simulink model "PID_Loop_2023a"  (R2023a)
settings: Solver=FixedStepAuto  StartTime=0.0  StopTime=tspan  FixedStep=dt  RelTol=1e-3
model workspace (MAT data in the model file):
  Drag_Constants = 1
  mass = [5.51 5.51 5.51 1 1 1]
  mass_6a = [5 5 5 1 1 1]
values from neighbouring files (symbols this model uses):
  do_bouyancy_flag = 1    [PID_testing_data_producer.m]    (also in init.m = 0)
  do_drag_flag = 1    [PID_testing_data_producer.m]
  do_gravity_flag = 1    [PID_testing_data_producer.m]    (also in init.m = 0)
  drag_wrench = [ ... (first row only)    [constants.m]    (also in constants.mat = [0.41 0 0 0 0 0 0 0.5 0 0 0 0 ... (36 elements, 6x6)])
  dt = 0.001    [PID_testing_data_producer.m]    (also in init.m)
  Dt = 0.01    [init.m]
  dt_controller = 0.01    [PID_testing_data_producer.m]
  dt_filter = 0.01    [PID_testing_data_producer.m]    (also in init.m)
  dt_imu = 0.01    [PID_testing_data_producer.m]
  dt_plotting = 0.01    [PID_testing_data_producer.m]
  g = 9.8067    [constants.m]    (also in constants.mat = 9.80665)
  H = [1 0 0 ... (first row only)    [init.m]
  inverse_wrench = pinv(wrench)    [calculate_wrench.m]    (also in constants.m = geometry_properties.inverse_wrench; geometry_properties.mat = [0.09 0.09 -0.09 -0.09 0.353553390593 0.353553390593 0.35355)
  max_pitch_torque = norm(wrench*(F_max*[1 1 -1 -1 0 0 0 0]'))    [calculate_wrench.m]
  max_roll_torque = norm(wrench*(F_max*[1 -1 1 -1 0 0 0 0]'))    [calculate_wrench.m]
  max_yaw_torque = norm(wrench*(F_max*[0 0 0 0 -1 1 -1 1]'))    [calculate_wrench.m]
  OperatingVoltage = Voltage    (= 16)    [constants.m]
  Q = diag([0.0001, 0.0001, 0.1])    [init.m]
  R = [.1 0 ... (first row only)    [init.m]
  states_desired = [x_des;E_des]    [init.m]
  v0_e = [0,0,0]'    [PID_testing_data_producer.m]    (also in init.m = [pi/6, -pi/6, pi]')
  Voltage = 16    [constants.m]
  volume = 0.0074    [constants.m]    (also in constants.mat = 0.0073741788)
  volume_center = [0, 0, -0.07]    [constants.m]    (also in constants.mat = [0 0 0.1])
  water_density = 997    [constants.m]    (also in constants.mat = 1000)
  waypoints = input_state_errors(:,i)    [PID_testing_data_producer.m]    (also in init.m = [0, 0, 0])
  wrench = eval(w)    [calculate_wrench.m]    (also in constants.m = geometry_properties.wrench; constants.mat = [0 0 0 0 -0.7071 -0.7071 -0.7071 -0.7071 0 0 0 0 ... (48 ele; geometry_properties.mat = [0 0 -1 0.22 0.25 0 0 0 -1 -0.22 0.25 0 ... (48 elements, 6x; wrench.m)
  x0_e = [0,0,0]'    [PID_testing_data_producer.m]    (also in init.m = [0, 0, 0]')
undefined symbols (not defined in the file or in its folder): IMU, P, Zero_Time
libraries: slpidlib x4, shared6dof x1, mspfiltlib x1, dspstat3 x1, mspsensorlib x1
(part 1 of 2)
settings Model: Creator=zenyn  LastModifiedBy=zafak
settings DataIOCC: LoggingToFile=on
settings OptimizationCC: EnhancedBackFolding=on  PassReuseOutputArgsAs=Individual arguments  ZeroExternalMemoryAtStartup=off  ZeroInternalMemoryAtStartup=off  MaxStackSize=64  OptimizeBlockOrder=speed  DifferentSizesBufferReuse=on  OptimizationCustomize=off  EfficientTunableParamExpr=on
settings DebuggingCC: ParameterTunabilityLossMsg=error
settings SFSimCC: MATLABDynamicMemAlloc=off
settings RTWCC: Description=Embedded Coder  SystemTargetFile=ert.tlc  HardwareBoard=Robot Operating System 2 (ROS 2)  TLCOptions="-aInlineSetEventsForThisBaseRateFcn=TLC_FALSE -aSuppressMultiTaskScheduler=TLC_FALSE  -aRateBasedStepFcn=0"  TemplateMakefile=ert_default_tmf  Toolchain=Colcon Tools  TargetLang=C++  GPUComputeCapability=5.0
settings CodeAppCC: ForceParamTrailComments=on  IgnoreCustomStorageClasses=off  OperatorAnnotations=on  SimulinkDataObjDesc=on  SFDataObjDesc=on  InsertBlockDesc=on
settings ERTTargetCC: CodeInterfacePackaging=C++ class  RootIOFormat=Structure reference

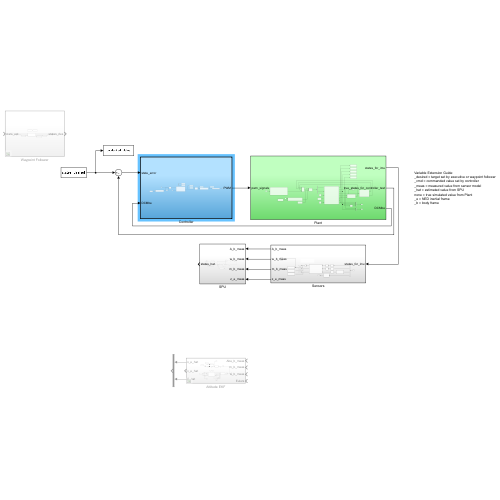
[thumbnail: Simulink's stored preview of the top-level diagram]
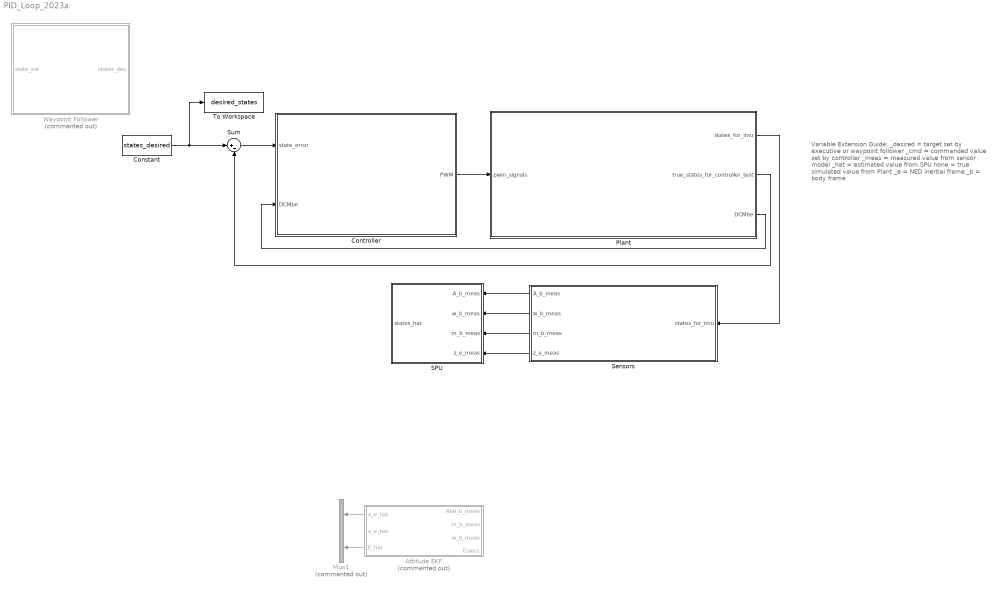
== system PID_Loop_2023a ==
  note: Variable Extension Guide:
      | _desired = target set by executive or waypoint follower
      | _cmd = commanded value set by controller
      | _meas = measured value from sensor model
      | _hat = estimated value from SPU
      | none = true simulated value from Plant
      | _e = NED inertial frame
      | _b = body frame
  Attitude EKF : Subsystem  Commented=on
  Constant : Constant  Value=states_desired
  Controller : Subsystem  TreatAsAtomicUnit=on
  Mux1 : Mux  Commented=on  Inputs=2
  Plant : Subsystem
  SPU : Subsystem
  Sensors : Subsystem
  Sum : Sum  Inputs=|+-
  To Workspace : ToWorkspace  VariableName=desired_states  SaveFormat=Timeseries  SampleTime=dt_plotting
  Waypoint Follower : Subsystem  Commented=on
  wires:
  Constant/1 -> Sum/1, To Workspace/1
  Sum/1 -> Controller/1(state_error)
  Controller/1(PWM) -> Plant/1(pwm_signals)
  Plant/2(true_states_for_controller_test) -> Sum/2
  Attitude EKF/1(x_e_hat) -> Mux1/1
  Attitude EKF/3(E_hat) -> Mux1/2
  Plant/1(states_for_imu) -> Sensors/1(states_for_imu)
  Sensors/1(A_b_meas) -> SPU/1(A_b_meas)
  Sensors/2(w_b_meas) -> SPU/2(w_b_meas)
  Sensors/3(m_b_meas) -> SPU/3(m_b_meas)
  Plant/3(DCMbe) -> Controller/2(DCMbe)
  Sensors/4(z_e_meas) -> SPU/4(z_e_meas)

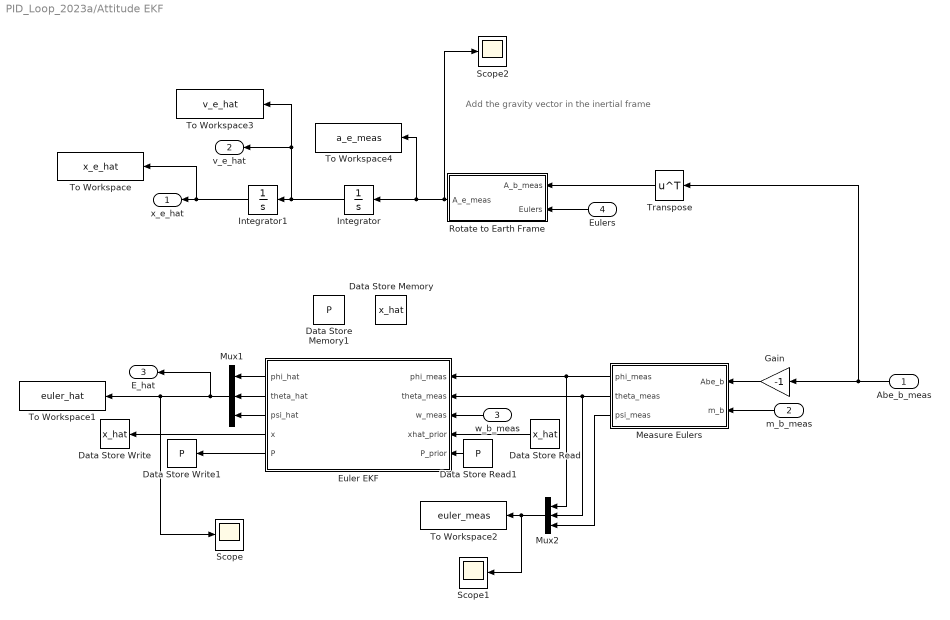
== system PID_Loop_2023a/Attitude EKF ==
  note: Add the gravity vector in the inertial frame
  Abe_b_meas : Inport  SampleTime=dt_filter
  m_b_meas : Inport  Port=2  SampleTime=dt_filter
  w_b_meas : Inport  Port=3
  Eulers : Inport  Port=4
  Data Store Memory : DataStoreMemory  DataStoreName=x_hat  WriteAfterWriteMsg=warning  InitialValue=xhat0  ShowAdditionalParam=off
  Data Store Memory1 : DataStoreMemory  DataStoreName=P  WriteAfterWriteMsg=warning  InitialValue=P0  ShowAdditionalParam=off
  Data Store Read : DataStoreRead  DataStoreName=x_hat  IndexOptions=Index vector (dialog)  Indices=1  OutputSizes=1
  Data Store Read1 : DataStoreRead  DataStoreName=P  IndexOptions=Index vector (dialog)  Indices=1  OutputSizes=1
  Data Store Write : DataStoreWrite  DataStoreName=x_hat  IndexOptions=Index vector (dialog)  Indices=1  OutputSizes=1
  Data Store Write1 : DataStoreWrite  DataStoreName=P  IndexOptions=Index vector (dialog)  Indices=1  OutputSizes=1
  Euler EKF : MATLAB Function  TreatAsAtomicUnit=on
  Gain : Gain  Gain=-1
  Integrator : Integrator  InitialCondition=v0_e
  Integrator1 : Integrator  InitialCondition=x0_e
  Measure Eulers : MATLAB Function  TreatAsAtomicUnit=on
  Mux1 : Mux  Inputs=3
  Mux2 : Mux  Inputs=3
  Rotate to Earth Frame : MATLAB Function  TreatAsAtomicUnit=on
  Scope : Scope
  Scope1 : Scope
  Scope2 : Scope
  To Workspace : ToWorkspace  VariableName=x_e_hat  SaveFormat=Timeseries  SampleTime=dt_plotting
  To Workspace1 : ToWorkspace  VariableName=euler_hat  SaveFormat=Timeseries  SampleTime=dt_plotting
  To Workspace2 : ToWorkspace  VariableName=euler_meas  SaveFormat=Timeseries  SampleTime=dt_plotting
  To Workspace3 : ToWorkspace  VariableName=v_e_hat  SaveFormat=Timeseries  SampleTime=dt_plotting
  To Workspace4 : ToWorkspace  VariableName=a_e_meas  SaveFormat=Timeseries  SampleTime=-1
  Transpose : Math  Operator=transpose
  x_e_hat : Outport
  v_e_hat : Outport  Port=2
  E_hat : Outport  Port=3
  wires:
  Measure Eulers/1(phi_meas) -> Euler EKF/1(phi_meas), Mux2/1
  Euler EKF/4(x) -> Data Store Write/1
  Measure Eulers/2(theta_meas) -> Mux2/2, Euler EKF/2(theta_meas)
  Mux1/1 -> E_hat/1, Scope/1, To Workspace1/1
  Data Store Read1/1 -> Euler EKF/5(P_prior)
  Euler EKF/1(phi_hat) -> Mux1/1
  Euler EKF/5(P) -> Data Store Write1/1
  Euler EKF/3(psi_hat) -> Mux1/3
  Euler EKF/2(theta_hat) -> Mux1/2
  Data Store Read/1 -> Euler EKF/4(xhat_prior)
  Abe_b_meas/1 -> Gain/1, Transpose/1
  Measure Eulers/3(psi_meas) -> Mux2/3
  Mux2/1 -> Scope1/1, To Workspace2/1
  m_b_meas/1 -> Measure Eulers/2(m_b)
  w_b_meas/1 -> Euler EKF/3(w_meas)
  Integrator/1 -> To Workspace3/1, v_e_hat/1, Integrator1/1
  Integrator1/1 -> To Workspace/1, x_e_hat/1
  Gain/1 -> Measure Eulers/1(Abe_b)
  Rotate to Earth Frame/1(A_e_meas) -> Scope2/1, To Workspace4/1, Integrator/1
  Eulers/1 -> Rotate to Earth Frame/2(Eulers)
  Transpose/1 -> Rotate to Earth Frame/1(A_b_meas)

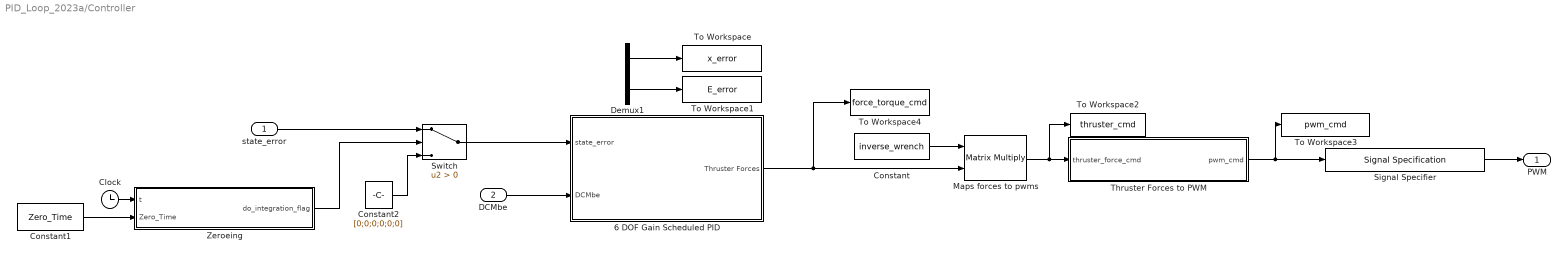
== system PID_Loop_2023a/Controller ==
  state_error : Inport  SampleTime=dt_controller
  DCMbe : Inport  Port=2
  6 DOF Gain Scheduled PID : Subsystem
  Clock : Clock
  Constant : Constant  Value=inverse_wrench
  Constant1 : Constant  Value=Zero_Time
  Constant2 : Constant  Value=[0;0;0;0;0;0]
  Demux1 : Demux  Outputs=2
  Maps forces to pwms : Product  Multiplication=Matrix(*)
  Signal Specifier : SignalSpecification  OutMin=[1200 ]  OutMax=[ 1800 ]  OutDataTypeStr=double  Unit=µs  Dimensions=[8 1]
  Switch : Switch  Criteria=u2 > Threshold  SaturateOnIntegerOverflow=off  InputSameDT=off
  Thruster Forces to PWM : MATLAB Function  TreatAsAtomicUnit=on
  To Workspace : ToWorkspace  VariableName=x_error  SaveFormat=Timeseries  SampleTime=dt_plotting
  To Workspace1 : ToWorkspace  VariableName=E_error  SaveFormat=Timeseries  SampleTime=dt_plotting
  To Workspace2 : ToWorkspace  VariableName=thruster_cmd  SaveFormat=Timeseries  SampleTime=dt_plotting
  To Workspace3 : ToWorkspace  VariableName=pwm_cmd  SaveFormat=Timeseries  SampleTime=dt_plotting
  To Workspace4 : ToWorkspace  VariableName=force_torque_cmd  SaveFormat=Timeseries  SampleTime=dt_plotting
  Zeroeing : MATLAB Function  TreatAsAtomicUnit=on
  PWM : Outport
  wires:
  Thruster Forces to PWM/1(pwm_cmd) -> Signal Specifier/1, To Workspace3/1
  Signal Specifier/1 -> PWM/1
  Demux1/1 -> To Workspace/1
  Demux1/2 -> To Workspace1/1
  Maps forces to pwms/1 -> Thruster Forces to PWM/1(thruster_force_cmd), To Workspace2/1
  Constant/1 -> Maps forces to pwms/1
  6 DOF Gain Scheduled PID/1(Thruster Forces) -> To Workspace4/1, Maps forces to pwms/2
  DCMbe/1 -> 6 DOF Gain Scheduled PID/2(DCMbe)
  Clock/1 -> Zeroeing/1(t)
  Constant1/1 -> Zeroeing/2(Zero_Time)
  Switch/1 -> 6 DOF Gain Scheduled PID/1(state_error)
  state_error/1 -> Switch/1
  Zeroeing/1(do_integration_flag) -> Switch/2
  Constant2/1 -> Switch/3

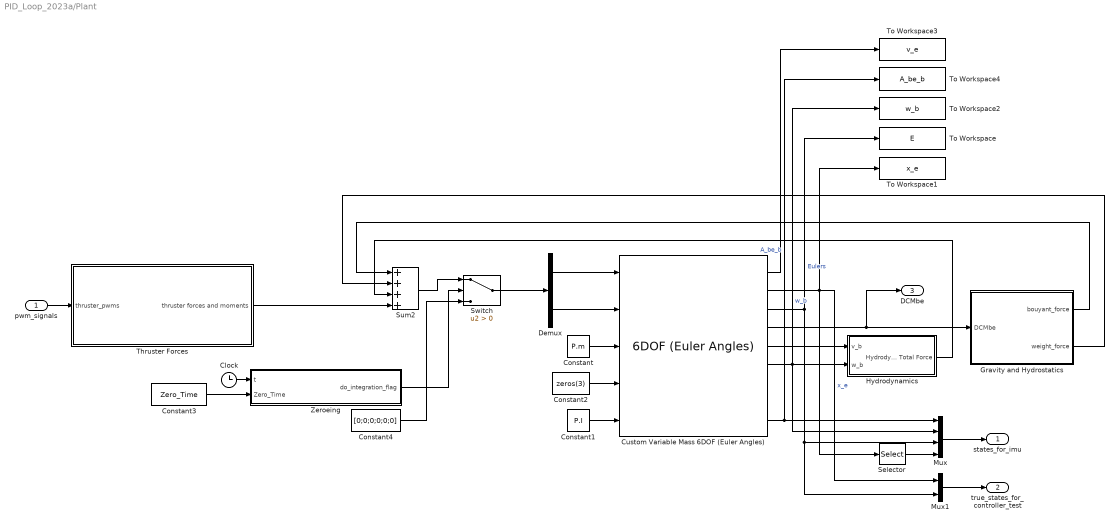
== system PID_Loop_2023a/Plant ==
  pwm_signals : Inport  SampleTime=dt
  Clock : Clock
  Constant : Constant  Value=P.m
  Constant1 : Constant  Value=P.I
  Constant2 : Constant  Value=zeros(3)
  Constant3 : Constant  Value=Zero_Time
  Constant4 : Constant  Value=[0;0;0;0;0;0]
  Custom Variable Mass 6DOF (Euler Angles) : shared6dof/6DOF (Euler Angles)  units=Metric (MKS)  mtype=Custom Variable  rep=Euler Angles  xme_0=x0_e  Vm_0=v0_e  eul_0=E0  pm_0=w0  mass_0=1.0  mass_e=0.5  mass_f=2.0  inertia=eye(3)  inertia_e=eye(3)  inertia_f=2*eye(3)  k_quat=1.0  vre_flag=off  abi_flag=on  aMode=0  xme_statename=''  Vm_statename=''  eul_statename=''  quat_statename=''  pm_statename=''  mass_statename=''
      settings: LibrarySourceBlock=aerolib6dof2/Custom Variable Mass 6DOF (Euler Angles)
  Demux : Demux  Outputs=2
  Gravity and Hydrostatics : Subsystem
  Hydrodynamics : Subsystem
  Mux : Mux
  Mux1 : Mux  Inputs=2
  Selector : Selector  InputPortWidth=3  IndexOptions=Index vector (dialog)  Indices=[3]  OutputSizes=1
  Sum2 : Sum  Inputs=++++
  Switch : Switch  Criteria=u2 > Threshold  SaturateOnIntegerOverflow=off  InputSameDT=off
  Thruster Forces : Subsystem
  To Workspace : ToWorkspace  VariableName=E  SaveFormat=Timeseries  SampleTime=dt_plotting
  To Workspace1 : ToWorkspace  VariableName=x_e  SaveFormat=Timeseries  SampleTime=dt_plotting
  To Workspace2 : ToWorkspace  VariableName=w_b  SaveFormat=Timeseries  SampleTime=dt_plotting
  To Workspace3 : ToWorkspace  VariableName=v_e  SaveFormat=Timeseries  SampleTime=dt_plotting
  To Workspace4 : ToWorkspace  VariableName=A_be_b  SaveFormat=Timeseries  SampleTime=dt_plotting
  Zeroeing : MATLAB Function  TreatAsAtomicUnit=on
  states_for_imu : Outport
  true_states_for_controller_test : Outport  Port=2
  DCMbe : Outport  Port=3
  wires:
  Constant/1 -> Custom Variable Mass 6DOF (Euler Angles)/3
  Constant1/1 -> Custom Variable Mass 6DOF (Euler Angles)/5
  Constant2/1 -> Custom Variable Mass 6DOF (Euler Angles)/4
  pwm_signals/1 -> Thruster Forces/1(thruster_pwms)
  Gravity and Hydrostatics/2(weight_force) -> Sum2/2
  Demux/2 -> Custom Variable Mass 6DOF (Euler Angles)/2
  Demux/1 -> Custom Variable Mass 6DOF (Euler Angles)/1
  Gravity and Hydrostatics/1(bouyant_force) -> Sum2/1
  Hydrodynamics/1(Hydrodynamic Total Force) -> Sum2/3
  Mux/1 -> states_for_imu/1
  Mux1/1 -> true_states_for_controller_test/1
  Custom Variable Mass 6DOF (Euler Angles)/4 -> DCMbe/1, Gravity and Hydrostatics/1(DCMbe)
  Custom Variable Mass 6DOF (Euler Angles)/5 -> Hydrodynamics/1(v_b)
  Custom Variable Mass 6DOF (Euler Angles)/6 -> Hydrodynamics/2(w_b), Mux/2, To Workspace2/1  "w_b"
  Custom Variable Mass 6DOF (Euler Angles)/9 -> To Workspace4/1, Mux/1  "A_be_b"
  Custom Variable Mass 6DOF (Euler Angles)/3 -> To Workspace/1, Mux1/2, Mux/3  "Eulers"
  Custom Variable Mass 6DOF (Euler Angles)/1 -> To Workspace3/1
  Thruster Forces/1(thruster forces and moments) -> Sum2/4
  Clock/1 -> Zeroeing/1(t)
  Constant3/1 -> Zeroeing/2(Zero_Time)
  Constant4/1 -> Switch/3
  Custom Variable Mass 6DOF (Euler Angles)/2 -> Mux1/1, Selector/1, To Workspace1/1  "x_e"
  Selector/1 -> Mux/4
  Sum2/1 -> Switch/1
  Switch/1 -> Demux/1
  Zeroeing/1(do_integration_flag) -> Switch/2

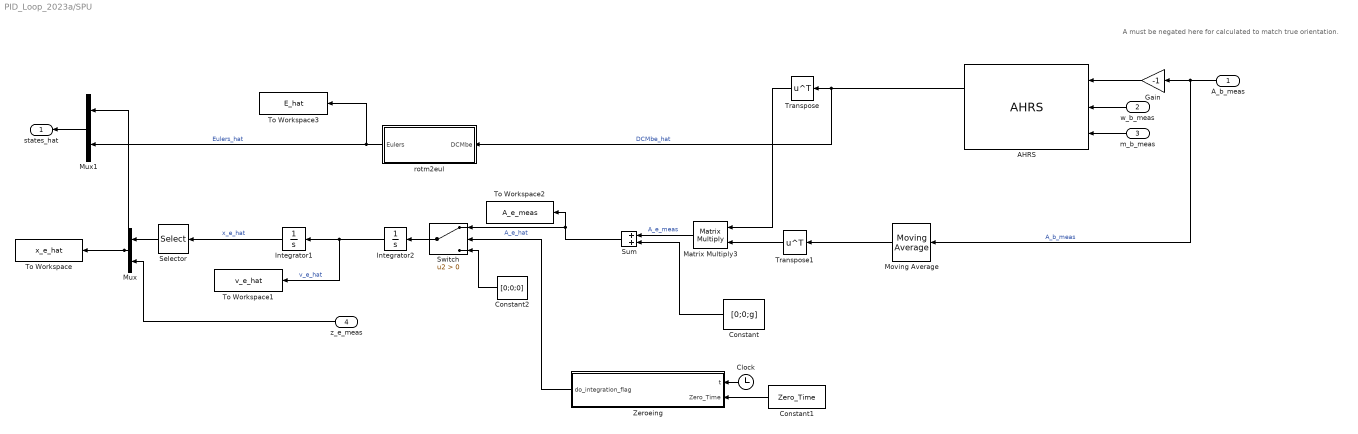
== system PID_Loop_2023a/SPU ==
  note: A must be negated here for calculated to match true orientation.
  A_b_meas : Inport  SampleTime=dt_filter
  w_b_meas : Inport  Port=2  SampleTime=dt_filter
  m_b_meas : Inport  Port=3  SampleTime=dt_filter
  z_e_meas : Inport  Port=4
  AHRS : mspfiltlib/AHRS  DispRefFrame=NED  DecimationFactor=1  InitialProcessNoise=ahrsfilter.defaultProcessNoise  OrientationFormat=Rotation matrix  SimulateUsing=Interpreted execution  AccelerometerNoise=AHRS.accel_noise  GyroscopeNoise=AHRS.gyro_noise  MagnetometerNoise=AHRS.mag_noise  GyroscopeDriftNoise=AHRS.gyro_drift_noise  LinearAccelerationNoise=AHRS.env_lin_accel_noise  MagneticDisturbanceNoise=AHRS.env_mag_disturbance_noise  LinearAccelerationDecayFactor=AHRS.env_lin_accel_decay_factor  MagneticDisturbanceDecayFactor=AHRS.env_mag_disturbance_decay_factor  ExpectedMagneticFieldStrength=AHRS.env_mag_field_strength
  Clock : Clock
  Constant : Constant  Value=[0;0;g]
  Constant1 : Constant  Value=Zero_Time
  Constant2 : Constant  Value=[0;0;0]
  Gain : Gain  Gain=-1
  Integrator1 : Integrator  InitialCondition=x0_e
  Integrator2 : Integrator  InitialCondition=v0_e
  Matrix Multiply3 : Product  Multiplication=Matrix(*)
  Moving Average : dspstat3/Moving Average  Method=Sliding window  ForgettingFactorPort=off  SpecifyWindowLength=on  WindowLength=10  OverlapLength=9  AllowArbitraryInputLength=off  ForgettingFactor=0.9  SimulateUsing=Code generation
  Mux : Mux  Inputs=2
  Mux1 : Mux  Inputs=2
  Selector : Selector  InputPortWidth=3  IndexOptions=Index vector (dialog)  Indices=[1 2]  OutputSizes=1
  Sum : Sum
  Switch : Switch  Criteria=u2 > Threshold  SaturateOnIntegerOverflow=off  InputSameDT=off
  To Workspace : ToWorkspace  VariableName=x_e_hat  SaveFormat=Timeseries  SampleTime=dt_plotting
  To Workspace1 : ToWorkspace  VariableName=v_e_hat  SaveFormat=Timeseries  SampleTime=dt_plotting
  To Workspace2 : ToWorkspace  VariableName=A_e_meas  SaveFormat=Timeseries  SampleTime=-1
  To Workspace3 : ToWorkspace  VariableName=E_hat  SaveFormat=Timeseries  SampleTime=-1
  Transpose : Math  Operator=transpose
  Transpose1 : Math  Operator=transpose
  Zeroeing : MATLAB Function  TreatAsAtomicUnit=on
  rotm2eul : MATLAB Function  TreatAsAtomicUnit=on
  states_hat : Outport
  wires:
  Mux/1 -> To Workspace/1, Mux1/1
  A_b_meas/1 -> Moving Average/1, Gain/1  "A_b_meas"
  Integrator2/1 -> To Workspace1/1, Integrator1/1  "v_e_hat"
  m_b_meas/1 -> AHRS/3
  AHRS/1 -> rotm2eul/1(DCMbe), Transpose/1  "DCMbe_hat"
  w_b_meas/1 -> AHRS/2
  Transpose/1 -> Matrix Multiply3/1
  Mux1/1 -> states_hat/1
  rotm2eul/1(Eulers) -> To Workspace3/1, Mux1/2  "Eulers_hat"
  Gain/1 -> AHRS/1
  Matrix Multiply3/1 -> Sum/1  "A_e_meas"
  Constant/1 -> Sum/2
  Transpose1/1 -> Matrix Multiply3/2
  Moving Average/1 -> Transpose1/1
  Clock/1 -> Zeroeing/1(t)
  Constant1/1 -> Zeroeing/2(Zero_Time)
  Constant2/1 -> Switch/3
  Integrator1/1 -> Selector/1  "x_e_hat"
  Selector/1 -> Mux/1
  Sum/1 -> To Workspace2/1, Switch/1  "A_e_hat"
  Switch/1 -> Integrator2/1
  z_e_meas/1 -> Mux/2
  Zeroeing/1(do_integration_flag) -> Switch/2

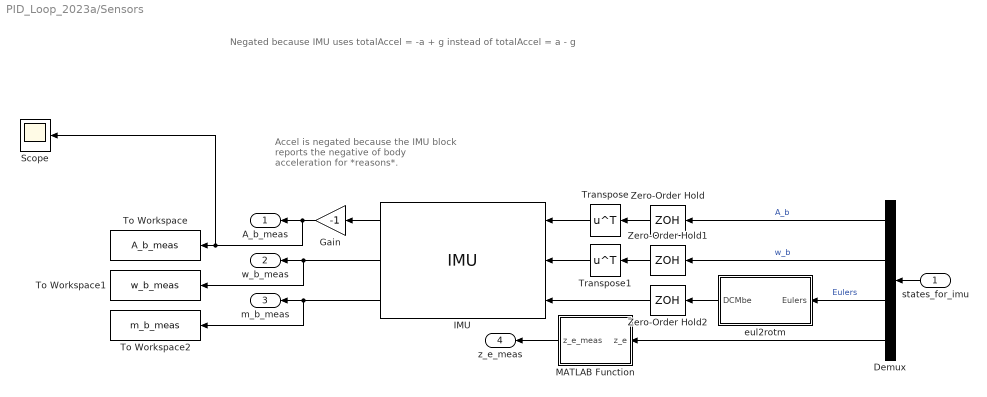
== system PID_Loop_2023a/Sensors ==
  note: Accel is negated because the IMU block reports the negative of body acceleration for *reasons*.
  note: Negated because IMU uses totalAccel = -a + g instead of totalAccel = a - g
  states_for_imu : Inport  SampleTime=dt_imu
  Demux : Demux  Outputs=[3,3,3,1]
  Gain : Gain  Gain=-1
  IMU : mspsensorlib/IMU  DispRefFrame=NED  Temperature=25  MagneticFieldNED=[27.550, -2.4169, -16]  MagneticFieldENU=[ -2.4169, 27.5550, 16.0849 ]  SeedDouble=102  SimulateUsing=Interpreted execution  AccelParamsMeasurementRange=IMU.accelMaxRating  AccelParamsResolution=0  AccelParamsConstantBias=[ 0, 0, 0 ]  AccelParamsAxesMisalignment=[ 100, 0, 0; 0, 100, 0; 0, 0, 100 ]  AccelParamsNoiseDensity=IMU.accelVelRNDWalk*[ 1, 1, 1 ]  AccelParamsBiasInstability=IMU.accelBiasInstability*[ 1, 1, 1 ]  AccelParamsRandomWalk=IMU.accelAccelRNDWalk*[1, 1, 1]  AccelParamsTemperatureBias=[ 0, 0, 0 ]  AccelParamsTemperatureScaleFactor=[ 0, 0, 0 ]  GyroParamsMeasurementRange=Inf  GyroParamsResolution=0  GyroParamsConstantBias=[ 0, 0, 0 ]  GyroParamsAxesMisalignment=[ 100, 0, 0; 0, 100, 0; 0, 0, 100 ]  GyroParamsAccelerationBias=[ 0, 0, 0 ]  GyroParamsNoiseDensity=IMU.gyroAngleRNDWalk*[ 1, 1, 1 ]  GyroParamsBiasInstability=IMU.gyroBiasInstability*[ 1, 1, 1 ]  GyroParamsRandomWalk=IMU.gyroRateRNDWalk*[1, 1, 1]  GyroParamsTemperatureBias=[ 0, 0, 0 ]  GyroParamsTemperatureScaleFactor=[ 0, 0, 0 ]  MagParamsMeasurementRange=Inf  MagParamsResolution=0  MagParamsConstantBias=[ 0, 0, 0 ]  MagParamsAxesMisalignment=[ 100, 0, 0; 0, 100, 0; 0, 0, 100 ]  MagParamsNoiseDensity=IMU.magsRateRNDWalk*[1, 1, 1]  MagParamsBiasInstability=IMU.magsBiasInstability*[1, 1, 1]  MagParamsRandomWalk=IMU.magsRNDWalk*[1, 1, 1]  MagParamsTemperatureBias=[ 0, 0, 0 ]  MagParamsTemperatureScaleFactor=[ 0, 0, 0 ]
  MATLAB Function : MATLAB Function  TreatAsAtomicUnit=on
  Scope : Scope
  To Workspace : ToWorkspace  VariableName=A_b_meas  SaveFormat=Timeseries  SampleTime=dt_plotting
  To Workspace1 : ToWorkspace  VariableName=w_b_meas  SaveFormat=Timeseries  SampleTime=dt_plotting
  To Workspace2 : ToWorkspace  VariableName=m_b_meas  SaveFormat=Timeseries  SampleTime=dt_plotting
  Transpose : Math  Operator=transpose
  Transpose1 : Math  Operator=transpose
  Zero-Order Hold : ZeroOrderHold  SampleTime=dt_filter
  Zero-Order Hold1 : ZeroOrderHold  SampleTime=dt_filter
  Zero-Order Hold2 : ZeroOrderHold  SampleTime=dt_filter
  eul2rotm : MATLAB Function  TreatAsAtomicUnit=on
  A_b_meas : Outport
  w_b_meas : Outport  Port=2
  m_b_meas : Outport  Port=3
  z_e_meas : Outport  Port=4
  wires:
  Transpose/1 -> IMU/1
  Zero-Order Hold/1 -> Transpose/1
  Transpose1/1 -> IMU/2
  Zero-Order Hold1/1 -> Transpose1/1
  Demux/1 -> Zero-Order Hold/1  "A_b"
  Zero-Order Hold2/1 -> IMU/3
  IMU/2 -> w_b_meas/1, To Workspace1/1
  IMU/3 -> m_b_meas/1, To Workspace2/1
  Demux/2 -> Zero-Order Hold1/1  "w_b"
  IMU/1 -> Gain/1
  Gain/1 -> Scope/1, To Workspace/1, A_b_meas/1
  states_for_imu/1 -> Demux/1
  Demux/3 -> eul2rotm/1(Eulers)  "Eulers"
  eul2rotm/1(DCMbe) -> Zero-Order Hold2/1
  Demux/4 -> MATLAB Function/1(z_e)
  MATLAB Function/1(z_e_meas) -> z_e_meas/1

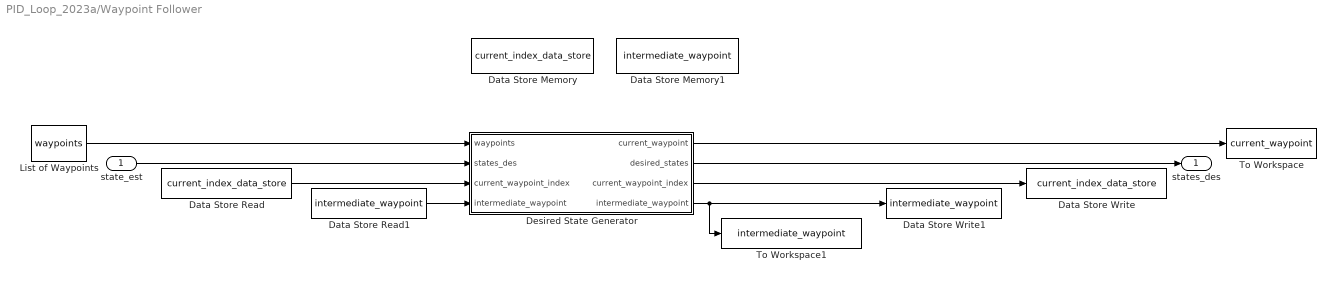
== system PID_Loop_2023a/Waypoint Follower ==
  state_est : Inport  SampleTime=Dt
  Data Store Memory : DataStoreMemory  DataStoreName=current_index_data_store  WriteAfterWriteMsg=warning  InitialValue=1  ShowAdditionalParam=off
  Data Store Memory1 : DataStoreMemory  DataStoreName=intermediate_waypoint  WriteAfterWriteMsg=warning  InitialValue=[9999,9999,9999]  ShowAdditionalParam=off
  Data Store Read : DataStoreRead  DataStoreName=current_index_data_store  IndexOptions=Index vector (dialog)  Indices=1  OutputSizes=1
  Data Store Read1 : DataStoreRead  DataStoreName=intermediate_waypoint  IndexOptions=Index vector (dialog)  Indices=1  OutputSizes=1
  Data Store Write : DataStoreWrite  DataStoreName=current_index_data_store  IndexOptions=Index vector (dialog)  Indices=1  OutputSizes=1
  Data Store Write1 : DataStoreWrite  DataStoreName=intermediate_waypoint  IndexOptions=Index vector (dialog)  Indices=1  OutputSizes=1
  Desired State Generator : MATLAB Function  TreatAsAtomicUnit=on
  List of Waypoints : Constant  Value=waypoints
  To Workspace : ToWorkspace  VariableName=current_waypoint  SaveFormat=Timeseries  SampleTime=-1
  To Workspace1 : ToWorkspace  VariableName=intermediate_waypoint  SaveFormat=Timeseries  SampleTime=-1
  states_des : Outport  SampleTime=Dt
  wires:
  state_est/1 -> Desired State Generator/2(states_des)
  Desired State Generator/2(desired_states) -> states_des/1
  Desired State Generator/3(current_waypoint_index) -> Data Store Write/1
  List of Waypoints/1 -> Desired State Generator/1(waypoints)
  Desired State Generator/1(current_waypoint) -> To Workspace/1
  Data Store Read/1 -> Desired State Generator/3("current_waypoint_index ")
  Data Store Read1/1 -> Desired State Generator/4("intermediate_waypoint ")
  Desired State Generator/4(intermediate_waypoint) -> Data Store Write1/1, To Workspace1/1

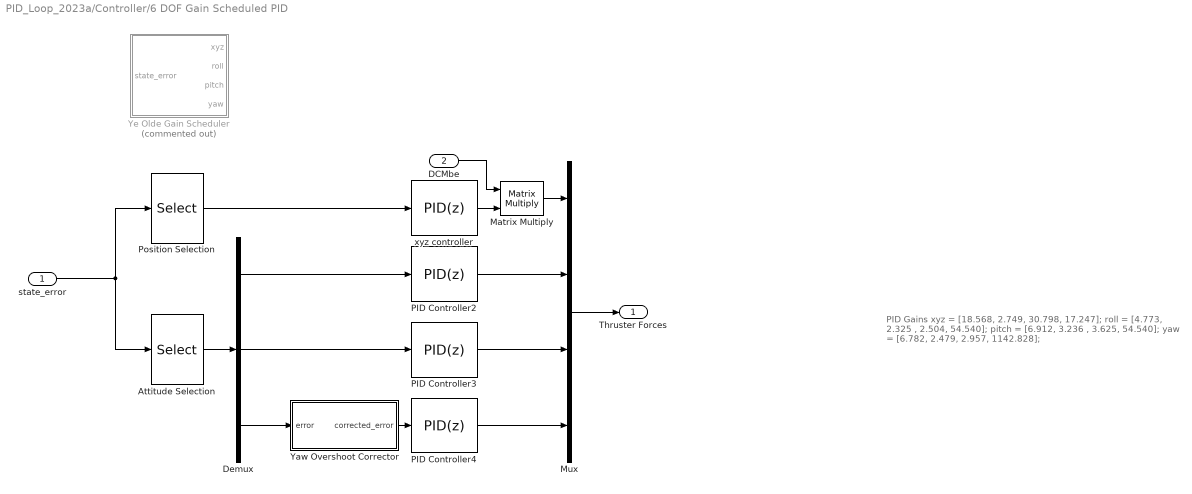
== system PID_Loop_2023a/Controller/6 DOF Gain Scheduled PID ==
  note: PID Gains
      |
      | xyz = [18.568, 2.749, 30.798, 17.247];
      | roll = [4.773, 2.325 , 2.504, 54.540];
      | pitch = [6.912, 3.236 , 3.625, 54.540];
      | yaw = [6.782, 2.479, 2.957, 1142.828];
  state_error : Inport  SampleTime=dt_controller
  DCMbe : Inport  Port=2
  Attitude Selection : Selector  InputPortWidth=6  IndexOptions=Index vector (dialog)  Indices=[4:6]  OutputSizes=1
  Demux : Demux  Outputs=3
  Matrix Multiply : Product  Multiplication=Matrix(*)
  Mux : Mux
  PID Controller2 : slpidlib/PID Controller  Controller=PID  Form=Parallel  TimeDomain=Discrete-time  UseExternalTs=off  SampleTime=-1  IntegratorMethod=Forward Euler  FilterMethod=Forward Euler  ControllerParametersSource=internal  P=4.773  I=2.325  UseKiTs=off  D=2.504  N=54.540  UseFilter=on  TunerSelectOption=Transfer Function Based (PID Tuner App)  InitialConditionSource=internal  InitialConditionForIntegrator=0  InitialConditionForFilter=0  DifferentiatorICPrevScaledInput=0  ExternalReset=none  TrackingMode=off  Kt=1  LimitOutput=on  SatLimitsSource=internal  UpperSaturationLimit=max_roll_torque  LowerSaturationLimit=-max_roll_torque  LinearizeAsGain=on  AntiWindupMode=none  Kb=1  LimitIntegrator=off  UpperIntegratorSaturationLimit=inf  LowerIntegratorSaturationLimit=-inf  POutMin=[]  POutMax=[]  IOutMin=[]  IOutMax=[]  DOutMin=[]  DOutMax=[]  NOutMin=[]  NOutMax=[]  SumOutMin=[]  SumOutMax=[]  SaturationOutMin=[]  SaturationOutMax=[]  PParamMin=[]  PParamMax=[]  IParamMin=[]  IParamMax=[]  DParamMin=[]  DParamMax=[]  NParamMin=[]  NParamMax=[]  KbParamMin=[]  KbParamMax=[]  KtParamMin=[]  KtParamMax=[]  KbOutMin=[]  KbOutMax=[]  KtOutMin=[]  KtOutMax=[]  IntegratorOutMin=[]  IntegratorOutMax=[]  FilterOutMin=[]  FilterOutMax=[]  SumI1OutMin=[]  SumI1OutMax=[]  SumI2OutMin=[]  SumI2OutMax=[]  SumI3OutMin=[]  SumI3OutMax=[]  SumI4OutMin=[]  SumI4OutMax=[]  SumDOutMin=[]  SumDOutMax=[]  DifferentiatorOutMin=[]  DifferentiatorOutMax=[]  FilterDiffOutCoefMin=[]  FilterDiffOutCoefMax=[]  ReciprocalOutMin=[]  ReciprocalOutMax=[]  SumDenOutMin=[]  SumDenOutMax=[]  SumNumOutMin=[]  SumNumOutMax=[]  DivideOutMin=[]  DivideOutMax=[]  UdiffTsProdOutMin=[]  UdiffTsProdOutMax=[]  NTsProdOutMin=[]  NTsProdOutMax=[]  UintegralTsProdOutMin=[]  UintegralTsProdOutMax=[]  UngainTsProdOutMin=[]  UngainTsProdOutMax=[]  ClampingZeroOutDataTypeStr=Inherit: Inherit via back propagation  ClampingZeroOutMin=[]  ClampingZeroOutMax=[]  FilterDenConstantOutDataTypeStr=Inherit: Inherit via back propagation  FilterDenConstantOutMin=[]  FilterDenConstantOutMax=[]  PCopyOutDataTypeStr=Inherit: Inherit via back propagation  PCopyOutMin=[]  PCopyOutMax=[]  NCopyOutDataTypeStr=Inherit: Inherit via back propagation  NCopyOutMin=[]  NCopyOutMax=[]  IntegratorContinuousStateAttributes=''  IntegratorStateMustResolveToSignalObject=off  IntegratorRTWStateStorageClass=Auto  FilterContinuousStateAttributes=''  FilterStateMustResolveToSignalObject=off  FilterRTWStateStorageClass=Auto  ParallelPVariant=InternalParameters  IdealPVariant=Disabled  IVariant=InternalParameters  DVariant=InternalParameters  IntegratorVariant=Discrete  SatVariant=Enabled  AWVariant=Passthrough  PCopyVariant=Disabled  TRVariant=Disabled  FdbkBlocksVariant=Forward  IdealPFdbkVariant=Disabled  SatFdbkVariant=Disabled  DerivativeFilterVariant=ForwardEulerFilter  NVariant=InternalParameters  NCopyVariant=Disabled  FilterICVariant=InternalICsFilter  IntegratorICVariant=InternalICs  ExternalResetVariant=Disabled  TRSumVariant=Passthrough  SumFdbkVariant=Disabled  SumVariant=Sum_PID  TsampFilterVariant=InternalTs  TsampNgainVariant=Passthrough  TsampIntegralVariant=Disabled_SignalSpec  ExternalSaturationOutDataTypeStr=Inherit: Same as second input
  PID Controller3 : slpidlib/PID Controller  Controller=PID  Form=Parallel  TimeDomain=Discrete-time  UseExternalTs=off  SampleTime=-1  IntegratorMethod=Forward Euler  FilterMethod=Forward Euler  ControllerParametersSource=internal  P=6.912  I=3.236  UseKiTs=off  D=3.625  N=54.540  UseFilter=on  TunerSelectOption=Transfer Function Based (PID Tuner App)  InitialConditionSource=internal  InitialConditionForIntegrator=0  InitialConditionForFilter=0  DifferentiatorICPrevScaledInput=0  ExternalReset=none  TrackingMode=off  Kt=1  LimitOutput=on  SatLimitsSource=internal  UpperSaturationLimit=max_pitch_torque  LowerSaturationLimit=-max_pitch_torque  LinearizeAsGain=on  AntiWindupMode=none  Kb=1  LimitIntegrator=off  UpperIntegratorSaturationLimit=inf  LowerIntegratorSaturationLimit=-inf  POutMin=[]  POutMax=[]  IOutMin=[]  IOutMax=[]  DOutMin=[]  DOutMax=[]  NOutMin=[]  NOutMax=[]  SumOutMin=[]  SumOutMax=[]  SaturationOutMin=[]  SaturationOutMax=[]  PParamMin=[]  PParamMax=[]  IParamMin=[]  IParamMax=[]  DParamMin=[]  DParamMax=[]  NParamMin=[]  NParamMax=[]  KbParamMin=[]  KbParamMax=[]  KtParamMin=[]  KtParamMax=[]  KbOutMin=[]  KbOutMax=[]  KtOutMin=[]  KtOutMax=[]  IntegratorOutMin=[]  IntegratorOutMax=[]  FilterOutMin=[]  FilterOutMax=[]  SumI1OutMin=[]  SumI1OutMax=[]  SumI2OutMin=[]  SumI2OutMax=[]  SumI3OutMin=[]  SumI3OutMax=[]  SumI4OutMin=[]  SumI4OutMax=[]  SumDOutMin=[]  SumDOutMax=[]  DifferentiatorOutMin=[]  DifferentiatorOutMax=[]  FilterDiffOutCoefMin=[]  FilterDiffOutCoefMax=[]  ReciprocalOutMin=[]  ReciprocalOutMax=[]  SumDenOutMin=[]  SumDenOutMax=[]  SumNumOutMin=[]  SumNumOutMax=[]  DivideOutMin=[]  DivideOutMax=[]  UdiffTsProdOutMin=[]  UdiffTsProdOutMax=[]  NTsProdOutMin=[]  NTsProdOutMax=[]  UintegralTsProdOutMin=[]  UintegralTsProdOutMax=[]  UngainTsProdOutMin=[]  UngainTsProdOutMax=[]  ClampingZeroOutDataTypeStr=Inherit: Inherit via back propagation  ClampingZeroOutMin=[]  ClampingZeroOutMax=[]  FilterDenConstantOutDataTypeStr=Inherit: Inherit via back propagation  FilterDenConstantOutMin=[]  FilterDenConstantOutMax=[]  PCopyOutDataTypeStr=Inherit: Inherit via back propagation  PCopyOutMin=[]  PCopyOutMax=[]  NCopyOutDataTypeStr=Inherit: Inherit via back propagation  NCopyOutMin=[]  NCopyOutMax=[]  IntegratorContinuousStateAttributes=''  IntegratorStateMustResolveToSignalObject=off  IntegratorRTWStateStorageClass=Auto  FilterContinuousStateAttributes=''  FilterStateMustResolveToSignalObject=off  FilterRTWStateStorageClass=Auto  ParallelPVariant=InternalParameters  IdealPVariant=Disabled  IVariant=InternalParameters  DVariant=InternalParameters  IntegratorVariant=Discrete  SatVariant=Enabled  AWVariant=Passthrough  PCopyVariant=Disabled  TRVariant=Disabled  FdbkBlocksVariant=Forward  IdealPFdbkVariant=Disabled  SatFdbkVariant=Disabled  DerivativeFilterVariant=ForwardEulerFilter  NVariant=InternalParameters  NCopyVariant=Disabled  FilterICVariant=InternalICsFilter  IntegratorICVariant=InternalICs  ExternalResetVariant=Disabled  TRSumVariant=Passthrough  SumFdbkVariant=Disabled  SumVariant=Sum_PID  TsampFilterVariant=InternalTs  TsampNgainVariant=Passthrough  TsampIntegralVariant=Disabled_SignalSpec  ExternalSaturationOutDataTypeStr=Inherit: Same as second input
  PID Controller4 : slpidlib/PID Controller  Controller=PID  Form=Parallel  TimeDomain=Discrete-time  UseExternalTs=off  SampleTime=-1  IntegratorMethod=Forward Euler  FilterMethod=Forward Euler  ControllerParametersSource=internal  P=6.782  I=2.479  UseKiTs=off  D=2.957  N=1142.828  UseFilter=on  TunerSelectOption=Transfer Function Based (PID Tuner App)  InitialConditionSource=internal  InitialConditionForIntegrator=0  InitialConditionForFilter=0  DifferentiatorICPrevScaledInput=0  ExternalReset=none  TrackingMode=off  Kt=1  LimitOutput=on  SatLimitsSource=internal  UpperSaturationLimit=max_yaw_torque  LowerSaturationLimit=-max_yaw_torque  LinearizeAsGain=on  AntiWindupMode=none  Kb=1  LimitIntegrator=off  UpperIntegratorSaturationLimit=inf  LowerIntegratorSaturationLimit=-inf  POutMin=[]  POutMax=[]  IOutMin=[]  IOutMax=[]  DOutMin=[]  DOutMax=[]  NOutMin=[]  NOutMax=[]  SumOutMin=[]  SumOutMax=[]  SaturationOutMin=[]  SaturationOutMax=[]  PParamMin=[]  PParamMax=[]  IParamMin=[]  IParamMax=[]  DParamMin=[]  DParamMax=[]  NParamMin=[]  NParamMax=[]  KbParamMin=[]  KbParamMax=[]  KtParamMin=[]  KtParamMax=[]  KbOutMin=[]  KbOutMax=[]  KtOutMin=[]  KtOutMax=[]  IntegratorOutMin=[]  IntegratorOutMax=[]  FilterOutMin=[]  FilterOutMax=[]  SumI1OutMin=[]  SumI1OutMax=[]  SumI2OutMin=[]  SumI2OutMax=[]  SumI3OutMin=[]  SumI3OutMax=[]  SumI4OutMin=[]  SumI4OutMax=[]  SumDOutMin=[]  SumDOutMax=[]  DifferentiatorOutMin=[]  DifferentiatorOutMax=[]  FilterDiffOutCoefMin=[]  FilterDiffOutCoefMax=[]  ReciprocalOutMin=[]  ReciprocalOutMax=[]  SumDenOutMin=[]  SumDenOutMax=[]  SumNumOutMin=[]  SumNumOutMax=[]  DivideOutMin=[]  DivideOutMax=[]  UdiffTsProdOutMin=[]  UdiffTsProdOutMax=[]  NTsProdOutMin=[]  NTsProdOutMax=[]  UintegralTsProdOutMin=[]  UintegralTsProdOutMax=[]  UngainTsProdOutMin=[]  UngainTsProdOutMax=[]  ClampingZeroOutDataTypeStr=Inherit: Inherit via back propagation  ClampingZeroOutMin=[]  ClampingZeroOutMax=[]  FilterDenConstantOutDataTypeStr=Inherit: Inherit via back propagation  FilterDenConstantOutMin=[]  FilterDenConstantOutMax=[]  PCopyOutDataTypeStr=Inherit: Inherit via back propagation  PCopyOutMin=[]  PCopyOutMax=[]  NCopyOutDataTypeStr=Inherit: Inherit via back propagation  NCopyOutMin=[]  NCopyOutMax=[]  IntegratorContinuousStateAttributes=''  IntegratorStateMustResolveToSignalObject=off  IntegratorRTWStateStorageClass=Auto  FilterContinuousStateAttributes=''  FilterStateMustResolveToSignalObject=off  FilterRTWStateStorageClass=Auto  ParallelPVariant=InternalParameters  IdealPVariant=Disabled  IVariant=InternalParameters  DVariant=InternalParameters  IntegratorVariant=Discrete  SatVariant=Enabled  AWVariant=Passthrough  PCopyVariant=Disabled  TRVariant=Disabled  FdbkBlocksVariant=Forward  IdealPFdbkVariant=Disabled  SatFdbkVariant=Disabled  DerivativeFilterVariant=ForwardEulerFilter  NVariant=InternalParameters  NCopyVariant=Disabled  FilterICVariant=InternalICsFilter  IntegratorICVariant=InternalICs  ExternalResetVariant=Disabled  TRSumVariant=Passthrough  SumFdbkVariant=Disabled  SumVariant=Sum_PID  TsampFilterVariant=InternalTs  TsampNgainVariant=Passthrough  TsampIntegralVariant=Disabled_SignalSpec  ExternalSaturationOutDataTypeStr=Inherit: Same as second input
  Position Selection : Selector  InputPortWidth=6  IndexOptions=Index vector (dialog)  Indices=[1:3]  OutputSizes=1
  Yaw Overshoot Corrector : MATLAB Function  TreatAsAtomicUnit=on
  Ye Olde Gain Scheduler : Subsystem  Commented=on
  xyz controller : slpidlib/PID Controller  Controller=PID  Form=Parallel  TimeDomain=Discrete-time  UseExternalTs=off  SampleTime=-1  IntegratorMethod=Forward Euler  FilterMethod=Forward Euler  ControllerParametersSource=internal  P=18.567926327114  I=2.74882046275699  UseKiTs=off  D=30.7980856287723  N=17.2469682941307  UseFilter=on  TunerSelectOption=Transfer Function Based (PID Tuner App)  InitialConditionSource=internal  InitialConditionForIntegrator=0  InitialConditionForFilter=0  DifferentiatorICPrevScaledInput=0  ExternalReset=none  TrackingMode=off  Kt=1  LimitOutput=on  SatLimitsSource=internal  UpperSaturationLimit=120  LowerSaturationLimit=-120  LinearizeAsGain=on  AntiWindupMode=none  Kb=1  LimitIntegrator=off  UpperIntegratorSaturationLimit=inf  LowerIntegratorSaturationLimit=-inf  POutMin=[]  POutMax=[]  IOutMin=[]  IOutMax=[]  DOutMin=[]  DOutMax=[]  NOutMin=[]  NOutMax=[]  SumOutMin=[]  SumOutMax=[]  SaturationOutMin=[]  SaturationOutMax=[]  PParamMin=[]  PParamMax=[]  IParamMin=[]  IParamMax=[]  DParamMin=[]  DParamMax=[]  NParamMin=[]  NParamMax=[]  KbParamMin=[]  KbParamMax=[]  KtParamMin=[]  KtParamMax=[]  KbOutMin=[]  KbOutMax=[]  KtOutMin=[]  KtOutMax=[]  IntegratorOutMin=[]  IntegratorOutMax=[]  FilterOutMin=[]  FilterOutMax=[]  SumI1OutMin=[]  SumI1OutMax=[]  SumI2OutMin=[]  SumI2OutMax=[]  SumI3OutMin=[]  SumI3OutMax=[]  SumI4OutMin=[]  SumI4OutMax=[]  SumDOutMin=[]  SumDOutMax=[]  DifferentiatorOutMin=[]  DifferentiatorOutMax=[]  FilterDiffOutCoefMin=[]  FilterDiffOutCoefMax=[]  ReciprocalOutMin=[]  ReciprocalOutMax=[]  SumDenOutMin=[]  SumDenOutMax=[]  SumNumOutMin=[]  SumNumOutMax=[]  DivideOutMin=[]  DivideOutMax=[]  UdiffTsProdOutMin=[]  UdiffTsProdOutMax=[]  NTsProdOutMin=[]  NTsProdOutMax=[]  UintegralTsProdOutMin=[]  UintegralTsProdOutMax=[]  UngainTsProdOutMin=[]  UngainTsProdOutMax=[]  ClampingZeroOutDataTypeStr=Inherit: Inherit via back propagation  ClampingZeroOutMin=[]  ClampingZeroOutMax=[]  FilterDenConstantOutDataTypeStr=Inherit: Inherit via back propagation  FilterDenConstantOutMin=[]  FilterDenConstantOutMax=[]  PCopyOutDataTypeStr=Inherit: Inherit via back propagation  PCopyOutMin=[]  PCopyOutMax=[]  NCopyOutDataTypeStr=Inherit: Inherit via back propagation  NCopyOutMin=[]  NCopyOutMax=[]  IntegratorContinuousStateAttributes=''  IntegratorStateMustResolveToSignalObject=off  IntegratorRTWStateStorageClass=Auto  FilterContinuousStateAttributes=''  FilterStateMustResolveToSignalObject=off  FilterRTWStateStorageClass=Auto  ParallelPVariant=InternalParameters  IdealPVariant=Disabled  IVariant=InternalParameters  DVariant=InternalParameters  IntegratorVariant=Discrete  SatVariant=Enabled  AWVariant=Passthrough  PCopyVariant=Disabled  TRVariant=Disabled  FdbkBlocksVariant=Forward  IdealPFdbkVariant=Disabled  SatFdbkVariant=Disabled  DerivativeFilterVariant=ForwardEulerFilter  NVariant=InternalParameters  NCopyVariant=Disabled  FilterICVariant=InternalICsFilter  IntegratorICVariant=InternalICs  ExternalResetVariant=Disabled  TRSumVariant=Passthrough  SumFdbkVariant=Disabled  SumVariant=Sum_PID  TsampFilterVariant=InternalTs  TsampNgainVariant=Passthrough  TsampIntegralVariant=Disabled_SignalSpec  ExternalSaturationOutDataTypeStr=Inherit: Same as second input
  Thruster Forces : Outport
  wires:
  state_error/1 -> Position Selection/1, Attitude Selection/1
  Attitude Selection/1 -> Demux/1
  Demux/3 -> Yaw Overshoot Corrector/1(error)
  Mux/1 -> Thruster Forces/1
  PID Controller2/1 -> Mux/2
  PID Controller3/1 -> Mux/3
  PID Controller4/1 -> Mux/4
  xyz controller/1 -> Matrix Multiply/2
  Matrix Multiply/1 -> Mux/1
  DCMbe/1 -> Matrix Multiply/1
  Position Selection/1 -> xyz controller/1
  Yaw Overshoot Corrector/1(corrected_error) -> PID Controller4/1
  Demux/2 -> PID Controller3/1
  Demux/1 -> PID Controller2/1

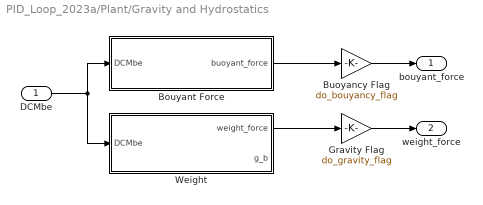
== system PID_Loop_2023a/Plant/Gravity and Hydrostatics ==
  DCMbe : Inport
  Bouyant Force : MATLAB Function  TreatAsAtomicUnit=on
  Buoyancy Flag : Gain  Gain=do_bouyancy_flag
  Gravity Flag : Gain  Gain=do_gravity_flag
  Weight : MATLAB Function  TreatAsAtomicUnit=on
  bouyant_force : Outport
  weight_force : Outport  Port=2
  wires:
  DCMbe/1 -> Weight/1(DCMbe), Bouyant Force/1(DCMbe)
  Buoyancy Flag/1 -> bouyant_force/1
  Gravity Flag/1 -> weight_force/1
  Weight/1(weight_force) -> Gravity Flag/1
  Bouyant Force/1(buoyant_force) -> Buoyancy Flag/1

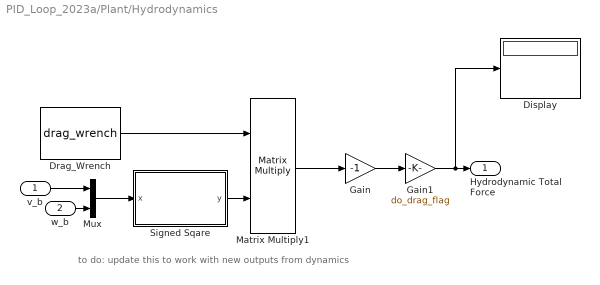
== system PID_Loop_2023a/Plant/Hydrodynamics ==
  note: to do: update this to work with new outputs from dynamics
  v_b : Inport
  w_b : Inport  Port=2
  Display : Display
  Drag_Wrench : Constant  Value=drag_wrench  VectorParams1D=off
  Gain : Gain  Gain=-1
  Gain1 : Gain  Gain=do_drag_flag
  Matrix Multiply1 : Product  Multiplication=Matrix(*)
  Mux : Mux  Inputs=2
  Signed Sqare : MATLAB Function  TreatAsAtomicUnit=on
  Hydrodynamic Total Force : Outport
  wires:
  Matrix Multiply1/1 -> Gain/1
  Drag_Wrench/1 -> Matrix Multiply1/1
  Signed Sqare/1(y) -> Matrix Multiply1/2
  Gain/1 -> Gain1/1
  Mux/1 -> Signed Sqare/1(x)
  v_b/1 -> Mux/1
  w_b/1 -> Mux/2
  Gain1/1 -> Display/1, Hydrodynamic Total Force/1

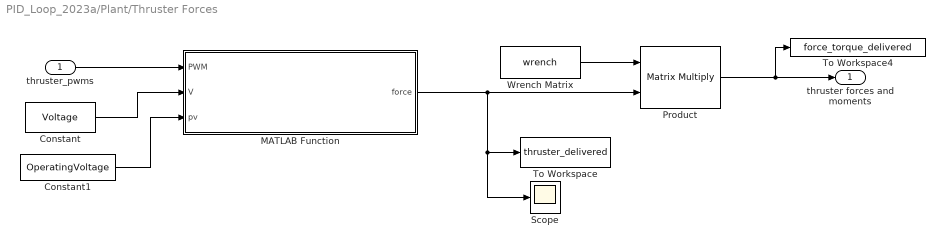
== system PID_Loop_2023a/Plant/Thruster Forces ==
  thruster_pwms : Inport  SampleTime=dt
  Constant : Constant  Value=Voltage
  Constant1 : Constant  Value=OperatingVoltage
  MATLAB Function : MATLAB Function  TreatAsAtomicUnit=on
  Product : Product  Multiplication=Matrix(*)
  Scope : Scope
  To Workspace : ToWorkspace  VariableName=thruster_delivered  SaveFormat=Timeseries  SampleTime=dt_plotting
  To Workspace4 : ToWorkspace  VariableName=force_torque_delivered  SaveFormat=Timeseries  SampleTime=dt_plotting
  Wrench Matrix : Constant  Value=wrench  VectorParams1D=off
  thruster forces and moments : Outport
  wires:
  Product/1 -> To Workspace4/1, thruster forces and moments/1
  thruster_pwms/1 -> MATLAB Function/1(PWM)
  Wrench Matrix/1 -> Product/1
  MATLAB Function/1(force) -> Product/2, Scope/1, To Workspace/1
  Constant/1 -> MATLAB Function/2(V)
  Constant1/1 -> MATLAB Function/3(pv)

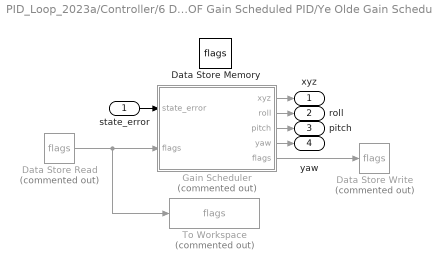
== system PID_Loop_2023a/Controller/6 DOF Gain Scheduled PID/Ye Olde Gain Scheduler ==
  state_error : Inport
  Data Store Memory : DataStoreMemory  DataStoreName=flags  WriteAfterWriteMsg=warning  InitialValue=[1 1 0]  ShowAdditionalParam=off
  Data Store Read : DataStoreRead  Commented=on  DataStoreName=flags  IndexOptions=Index vector (dialog)  Indices=1  OutputSizes=1
  Data Store Write : DataStoreWrite  Commented=on  DataStoreName=flags  IndexOptions=Index vector (dialog)  Indices=1  OutputSizes=1
  Gain Scheduler : MATLAB Function  Commented=on  TreatAsAtomicUnit=on
  To Workspace : ToWorkspace  Commented=on  VariableName=flags  SaveFormat=Timeseries  SampleTime=dt_plotting
  xyz : Outport
  roll : Outport  Port=2
  pitch : Outport  Port=3
  yaw : Outport  Port=4
  wires:
  state_error/1 -> Gain Scheduler/1(state_error)
  Gain Scheduler/2(roll) -> roll/1
  Data Store Read/1 -> To Workspace/1, Gain Scheduler/2("flags ")
  Gain Scheduler/1(xyz) -> xyz/1
  Gain Scheduler/5(flags) -> Data Store Write/1
  Gain Scheduler/3(pitch) -> pitch/1
  Gain Scheduler/4(yaw) -> yaw/1

== matlab function PID_Loop_2023a/SPU/rotm2eul ==
  data: DCMbe input; Eulers output
function Eulers = fcn(DCMbe)

Eulers = rotm2eul(DCMbe)';
%[Z Y X] by default
Eulers = [Eulers(3);Eulers(2);Eulers(1)];

== matlab function PID_Loop_2023a/Attitude EKF/Measure Eulers ==
  data: phi_meas output; Abe_b input; theta_meas output; m_b input; psi_meas output
function [phi_meas, theta_meas, psi_meas] = fcn(Abe_b,m_b)

%This function calculates the attitude of the vehicle using the
%acceleration vector direction and the magnetic field vector direction
%based on the assumption that the only acceleration is gravity in the
%inertial up (+z) direction and the magnetic field points in the inertial north
%(+x).

%unpack input
ax = Abe_b(1);
ay = Abe_b(2);
az = Abe_b(3);
mx = m_b(1);
my = m_b(2);


theta_meas = atan2((-ax), sqrt(ay*ay + az*az));
phi_meas = atan2(ay,az);
psi_meas = atan2(-my, mx);

== matlab function PID_Loop_2023a/Controller/6 DOF Gain Scheduled PID/Ye Olde Gain Scheduler/Gain Scheduler ==
  data: state_error input; xyz output; roll output; pitch output; yaw output; flags input; flags output
%The goal is to take state errors, determine the most desired state which
%we want to control. And then determine the gains to optimize that state
%control.

% If(roll error > Some saturation value)

%Yaw should have a much smaller error for this code architecture, we want
%to be pretty accurate

function[xyz, roll, pitch, yaw,flags] = gainScheduler(state_error,flags)

%unpack flags
roll_flag = flags(1);
pitch_flag = flags(2);
yaw_flag = flags(3);

roll_err = state_error(4); %Phi
pitch_err = state_error(5); %Theta
yaw_err = state_error(6); %Psi

%% Upper and Lower error bounds for control

%gain scheduling parameters
roll_upper = 5*pi/180;
roll_lower = 1*pi/180;
pitch_upper = 5*pi/180;
pitch_lower = 1*pi/180;
yaw_upper = 5*pi/180;
yaw_lower = 1*pi/180;




%% Roll, Pitch, and Yaw Flaggers
if(abs(yaw_err) >= yaw_upper)
    yaw_flag = 1;
elseif(abs(yaw_err) < yaw_lower)
    yaw_flag = 0;
else
    yaw_flag = yaw_flag;
end

if(abs(pitch_err) >= pitch_upper)
    pitch_flag = 1;
    yaw_flag = 0;
elseif(abs(pitch_err) < pitch_lower)
    pitch_flag = 0;
else
    pitch_flag = pitch_flag;
    if(pitch_flag == 1)
        yaw_flag = 0;
    end
end

if(abs(roll_err) >= roll_upper)
    roll_flag = 1;
    yaw_flag = 0;
elseif(abs(roll_err) < roll_lower)
    roll_flag = 0;
else
    roll_flag = roll_flag;
    if(roll_flag == 1)
        yaw_flag = 0;
    end
end


%% Scheduler


%Roll, Pitch, and Yaw Scheduling
if((roll_flag == 1) || (pitch_flag == 1))
    %don't want position and yaw control here
    roll = [4.773, 2.325 , 2.504, 54.540];
    pitch = [6.912, 3.236 , 3.625, 54.540];
    yaw = 1*[6.782, 2.479, 2.957, 1142.828];
    xyz = 1*[18.568, 2.749, 30.798, 17.247];
elseif(yaw_flag == 1)
    %do yaw control if pitch and roll are ok
    yaw = [6.782, 2.479, 2.957, 1142.828];
    roll = [4.773, 2.325 , 2.504, 54.540];
    pitch = [6.912, 3.236 , 3.625, 54.540];
    xyz = 1*[18.568, 2.749, 30.798, 17.247];
  

else
    %do position control, ok to leave on roll pitch and yaw because error
    %should be small
    xyz = [18.568, 2.749, 30.798, 17.247];
    roll = [4.773, 2.325 , 2.504, 54.540];
    pitch = [6.912, 3.236 , 3.625, 54.540];
    yaw = [6.782, 2.479, 2.957, 1142.828];
    
end

%pack up flags
flags = [roll_flag,pitch_flag,yaw_flag]';
end

== matlab function PID_Loop_2023a/Sensors/MATLAB Function ==
  data: z_e input; z_e_meas output
function z_e_meas = fcn(z_e)

z_e_meas = z_e;

== matlab function PID_Loop_2023a/Controller/6 DOF Gain Scheduled PID/Yaw Overshoot Corrector ==
  data: error input; corrected_error output
function corrected_error = fcn(error)
    if(error > 180)
        corrected_error = error - 360;
    elseif(error < -180)
        corrected_error = error + 360;
    else
        corrected_error = error;
    end
end

== matlab function PID_Loop_2023a/Attitude EKF/Rotate to Earth Frame ==
  data: A_b_meas input; A_e_meas output; Eulers input
function A_e_meas= fcn(A_b_meas,Eulers)
DCMbe = eul2rotm([Eulers(3),Eulers(2),Eulers(1)]);
A_e_meas = DCMbe*A_b_meas + [0;0;9.81];

== matlab function PID_Loop_2023a/SPU/Zeroeing ==
  data: t input; do_integration_flag output; Zero_Time input
function do_integration_flag = fcn(t,Zero_Time)

if(t < Zero_Time)
    do_integration_flag = 0;
else
    do_integration_flag = 1;
end

== matlab function PID_Loop_2023a/Plant/Zeroeing ==
  data: t input; do_integration_flag output; Zero_Time input
function do_integration_flag = fcn(t,Zero_Time)

if(t < Zero_Time)
    do_integration_flag = 0;
else
    do_integration_flag = 1;
end

== matlab function PID_Loop_2023a/Controller/Zeroeing ==
  data: t input; do_integration_flag output; Zero_Time input
function do_integration_flag = fcn(t,Zero_Time)

if(t < Zero_Time)
    do_integration_flag = 0;
else
    do_integration_flag = 1;
end

== matlab function PID_Loop_2023a/Plant/Hydrodynamics/Signed Sqare ==
  data: x input; y output
function y = signed_square(x)
y = x .* abs(x);
end

== matlab function PID_Loop_2023a/Plant/Thruster Forces/MATLAB Function ==
  data: PWM input size=8 [1099..1901]; V input; pv input; force output size=8 [-100..100]
function force = ForceFromPWMVoltage(PWM, V, pv)
    
%Set Main Operating Voltage to Determine Zero Band Used

% Clip PWM between 1100 and 1900
    PWM = min(max(PWM, 1100), 1900);

    % Offset PWM
    P = PWM - 1500;

    % Initialize force
    force = zeros(size(PWM));      % centre band defaults to 0

    if pv < 16
        lowBand  = -40;   highBand =  40;
    
        % lower band
        idx_l = (P <= lowBand);
        if any(idx_l)
            Pl = P(idx_l);   Vl = V;
            force(idx_l) = 9.80665*(...
                 0.18450859598294592 + ...
                -0.03877245224750089 * Vl + ...
                 0.00437326839182978 * Vl.^2 + ...
                -0.00014159192815009454 * Vl.^3 + ...
                 0.0047430745735151875 * Pl + ...
                -0.0011779727652119001 * Pl .* Vl + ...
                 0.00012626694389350853 * Pl .* Vl.^2 + ...
                -3.6521719807495034e-06 * Pl .* Vl.^3 + ...
                -3.394361152608232e-05 * Pl.^2 + ...
                 7.081135717273334e-06 * Pl.^2 .* Vl + ...
                -6.937006893095161e-07 * Pl.^2 .* Vl.^2 + ...
                 1.7574133886452198e-08 * Pl.^2 .* Vl.^3 + ...
                -1.0125491849106606e-07 * Pl.^3 + ...
                 2.3956832126051456e-08 * Pl.^3 .* Vl + ...
                -2.0262771883546578e-09 * Pl.^3 .* Vl.^2 + ...
                 5.312516822050221e-11 * Pl.^3 .* Vl.^3);
        end
    
        % upper band
        idx_u = (P >= highBand);
        if any(idx_u)
            Pu = P(idx_u);   Vu = V;
            force(idx_u) = 9.80665*(...
                -2.2103591356566494 + ...
                 0.5020761226661944 * Vu + ...
                -0.038894245021323104 * Vu.^2 + ...
                 0.0009685515042413979 * Vu.^3 + ...
                 0.04287528029632993 * Pu + ...
                -0.010018667907150527 * Pu .* Vu + ...
                 0.0007918978226055346 * Pu .* Vu.^2 + ...
                -1.965296626711245e-05 * Pu .* Vu.^3 + ...
                -0.00015245579360787697 * Pu.^2 + ...
                 3.5803548508328624e-05 * Pu.^2 .* Vu + ...
                -2.3976087919487086e-06 * Pu.^2 .* Vu.^2 + ...
                 5.395703879569961e-08 * Pu.^2 .* Vu.^3 + ...
                 1.3322303527138988e-07 * Pu.^3 + ...
                -2.9258256623955067e-08 * Pu.^3 .* Vu + ...
                 1.7469073167777621e-09 * Pu.^3 .* Vu.^2 + ...
                -3.0349724016130765e-11 * Pu.^3 .* Vu.^3);
        end
    
    % == HIGH-SUPPLY FAMILY (pv ≥ 16) ==============================
    else
        lowBand  = -28;   highBand =  28;
    
        % lower band
        idx_l = (P <= lowBand);
        if any(idx_l)
            Pl = P(idx_l);   Vl = V;
            force(idx_l) = 9.80665*(...
                 0.08254487160555046 + ...
                -0.019480220675947152 * Vl + ...
                 0.0028936369449359288 * Vl.^2 + ...
                -0.00010138307572005322 * Vl.^3 + ...
                 0.003229898558180788 * Pl + ...
                -0.0008968265330310558 * Pl .* Vl + ...
                 0.00010465994797731376 * Pl .* Vl.^2 + ...
                -3.055535261088971e-06 * Pl .* Vl.^3 + ...
                -4.055726784727783e-05 * Pl.^2 + ...
                 8.295219187479552e-06 * Pl.^2 .* Vl + ...
                -7.871417820116173e-07 * Pl.^2 .* Vl.^2 + ...
                 2.018189374507016e-08 * Pl.^2 .* Vl.^3 + ...
                -1.1008626859765426e-07 * Pl.^3 + ...
                 2.5564298545331497e-08 * Pl.^3 .* Vl + ...
                -2.150125796817501e-09 * Pl.^3 .* Vl.^2 + ...
                 5.66075567906357e-11 * Pl.^3 .* Vl.^3);
        end
    
        % upper band
        idx_u = (P >= highBand);
        if any(idx_u)
            Pu = P(idx_u);   Vu = V;
            force(idx_u) = 9.80665*(...
                -1.301472592175583 + ...
                 0.29936256569217357 * Vu + ...
                -0.023862645553737804 * Vu.^2 + ...
                 0.000604424709842914 * Vu.^3 + ...
                 0.028430427283555017 * Pu + ...
                -0.006798999839840506 * Pu .* Vu + ...
                 0.0005532577424440186 * Pu .* Vu.^2 + ...
                -1.386998112663601e-05 * Pu .* Vu.^3 + ...
                -8.657617313618081e-05 * Pu.^2 + ...
                 2.1124768936001382e-05 * Pu.^2 .* Vu + ...
                -1.3098984819064634e-06 * Pu.^2 .* Vu.^2 + ...
                 2.7592710221785262e-08 * Pu.^2 .* Vu.^3 + ...
                 4.2685499993615604e-08 * Pu.^3 + ...
                -9.090161175851121e-09 * Pu.^3 .* Vu + ...
                 2.5267430874260785e-10 * Pu.^3 .* Vu.^2 + ...
                 5.873211599828194e-12 * Pu.^3 .* Vu.^3);
        end
    end
    end

== matlab function PID_Loop_2023a/Sensors/eul2rotm ==
  data: Eulers input; DCMbe output
function DCMbe = fcn(Eulers)

DCMbe = eul2rotm([Eulers(3), Eulers(2), Eulers(1)]);

== matlab function PID_Loop_2023a/Controller/Thruster Forces to PWM ==
  data: thruster_force_cmd input; pwm_cmd output
function pwm_cmd = fcn(thruster_force_cmd)

pwm_cmd = zeros(8,1);
%uses a curve fit for thrust to pwm from the t200 thruster data sheet

for i=1:length(pwm_cmd)
    x = thruster_force_cmd(i);
    y = 0;

    if(x>0)
        y = round(0.00231011300235566*x^3 + -0.229204832763592*x^2 + 13.7272237851422*x + 1536.34500151024);
    elseif(x<0)
        y = round(0.00475737746846442*x^3 + 0.360062809963915*x^2 + 17.2034080439155*x + 1463.91061014397);
    else
        y = 1500;
    end

    %saturation
    if(y > 1900)
        y = 1900;
    end
    if (y < 1100)
        y = 1100;
    end

    pwm_cmd(i) = y;

end
